simulink model "HumanDynamicsTest"  (R2021b)
settings: Solver=ode3  StartTime=0.0  StopTime=20  FixedStep=Ts  RelTol=1e-3
values from neighbouring files (symbols this model uses):
  B_m = diag(ones(1,dh.dof)) * 32    [setup_teleop.m]
  gravity = [0 0 9.81]'    [setup_robot.m]
  K_m = diag(ones(1,dh.dof)) * 22    [setup_teleop.m]
  KD_h = eye(dh.dof_task) * 2*z*wn    [setup_teleop.m]
  KP_h = eye(dh.dof_task) * wn^2    [setup_teleop.m]
  M_m = diag(ones(1,dh.dof)) * 22    [setup_teleop.m]
undefined symbols (not defined in the file or in its folder): conf, dh, Fm_A, Fm_B, x0
libraries: robotcorelib x1, simulink x1
settings Model: Creator=Sebastiano  LastModifiedBy=Sebastiano

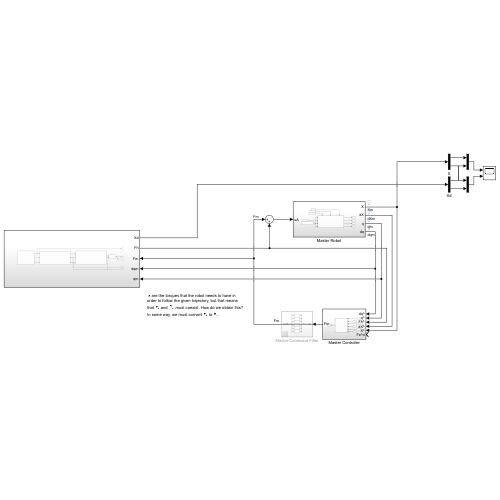
[thumbnail: Simulink's stored preview of the top-level diagram]
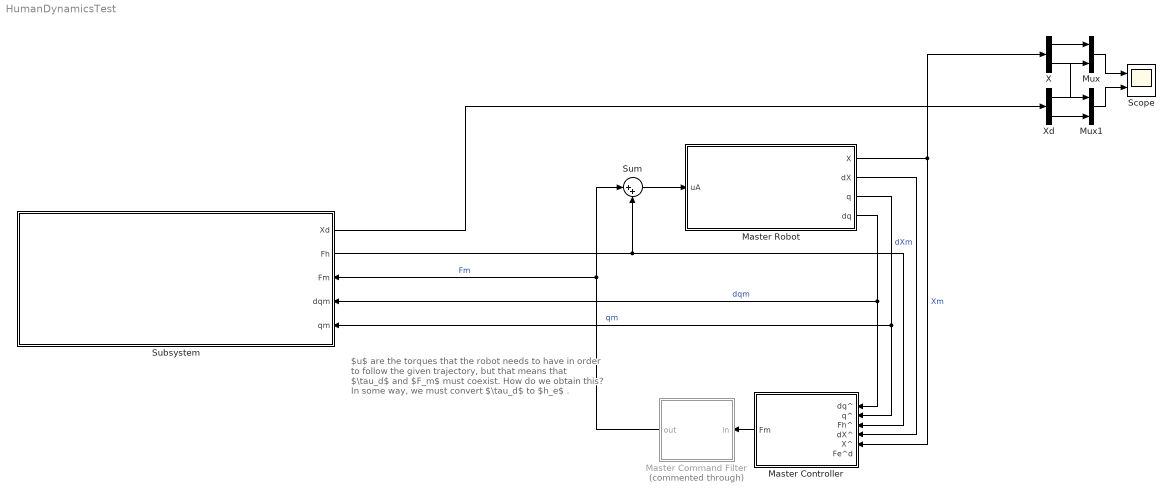
== system HumanDynamicsTest ==
  note: $u$ are the torques that the robot needs to have in order to follow the given trajectory, but that means that $\tau_d$ and $F_m$ must coexist. How do we obtain this? In some way, we must convert $\tau_d$ to $h_e$ .
  Master Command Filter : Subsystem  Commented=through
  Master Controller : Subsystem
  Master Robot : Subsystem
  Mux : Mux  Inputs=2
  Mux1 : Mux  Inputs=2
  Scope : Scope  NumInputPorts=2
  Subsystem : Subsystem
      settings: PortSchema="{\"entries\":[{\"content\":{\"sides\":[{\"content\":{\"connectorIds\":[]},\"type\":\"ConnectorPlacement.EquallySpacedRectSide\",\"uuid\":\"7778f5b7-85d4-4afc-857c-056ec77f7c35\"},{\"content\":{\"connectorIds\":[\"Out1\",\"Out2\",\"In1\",\"In2\",\"In3\"],\"side\":\"RIGHT\"},\"type\":\"ConnectorPlacement.EquallySpacedRectSide\",\"uuid\":\"4e6a4d83-f8e8-4554-84b1-926a6f2c9c17\"},{\"content\":{\"connectorIds\":[],\"side\":\"TOP\"},\"type\":\"ConnectorPlacement.EquallySpacedRectSide\",\"uuid\":\"7c53f63a-15b9-4620-895a-15c4690edfa5\"}]},\"type\":\"ConnectorPlacement.EquallySpacedConnector\",\"uuid\":\"f47fbd83-fa7b-4372-bf8b-e8c7b2e83c33\"}],\"packageUris\":[\"http://schema.mathworks.com/mf0/Connector/R2020b\"],\"version\":\"1.0\"}"
  Sum : Sum  Inputs=|++
  X : Demux  Outputs=2
  Xd : Demux  Outputs=2
  wires:
  Master Robot/3(q) -> Master Controller/2(q^), Subsystem/3(qm)  "qm"
  Master Robot/4(dq) -> Master Controller/1(dq^), Subsystem/2(dqm)  "dqm"
  Master Controller/1(Fm) -> Master Command Filter/1(in)
  Sum/1 -> Master Robot/1(uA)
  Master Robot/1(X) -> X/1, Master Controller/5(X^)  "Xm"
  Master Robot/2(dX) -> Master Controller/4(dX^)  "dXm"
  X/1 -> Mux/1
  Xd/1 -> Mux/2
  X/2 -> Mux1/1
  Xd/2 -> Mux1/2
  Mux/1 -> Scope/1
  Mux1/1 -> Scope/2
  Master Command Filter/1(out) -> Sum/1, Subsystem/1(Fm)  "Fm"
  Subsystem/2(Fh) -> Sum/2, Master Controller/3(Fh^)
  Subsystem/1(Xd) -> Xd/1

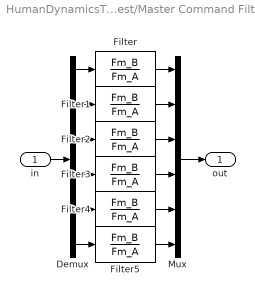
== system HumanDynamicsTest/Master Command Filter ==
  in : Inport
  Demux : Demux  Outputs=6
  Filter{,1..5} (6 alike) : TransferFcn  Numerator=Fm_B  Denominator=Fm_A
  Mux : Mux  Inputs=6
  out : Outport
  wires:
  Demux/4 -> Filter3/1
  Demux/6 -> Filter5/1
  Demux/2 -> Filter1/1
  Demux/5 -> Filter4/1
  Demux/1 -> Filter/1
  Demux/3 -> Filter2/1
  in/1 -> Demux/1
  Mux/1 -> out/1
  Filter/1 -> Mux/1
  Filter1/1 -> Mux/2
  Filter2/1 -> Mux/3
  Filter3/1 -> Mux/4
  Filter4/1 -> Mux/5
  Filter5/1 -> Mux/6

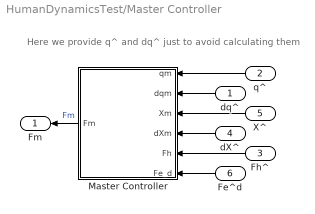
== system HumanDynamicsTest/Master Controller ==
  note: Here we provide q^ and dq^ just to avoid calculating them
  dq^ : Inport
  q^ : Inport  Port=2
  Fh^ : Inport  Port=3
  dX^ : Inport  Port=4
  X^ : Inport  Port=5
  Fe^d : Inport  Port=6
  Master Controller : MATLAB Function  TreatAsAtomicUnit=on
  Fm : Outport
  wires:
  Fh^/1 -> Master Controller/5(Fh)
  Fe^d/1 -> Master Controller/6(Fe_d)
  Master Controller/1(Fm) -> Fm/1  "Fm"
  X^/1 -> Master Controller/3(Xm)
  dX^/1 -> Master Controller/4(dXm)
  dq^/1 -> Master Controller/2(dqm)
  q^/1 -> Master Controller/1(qm)

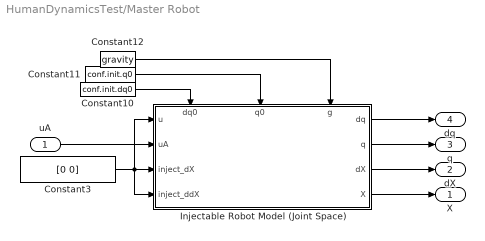
== system HumanDynamicsTest/Master Robot ==
  uA : Inport
  Constant10 : Constant  Value=conf.init.dq0
  Constant11 : Constant  Value=conf.init.q0
  Constant12 : Constant  Value=gravity
  Constant3 : Constant  Value=[0 0]
  Injectable Robot Model (Joint Space) : Subsystem
      settings: PortSchema="{\"entries\":[{\"content\":{\"sides\":[{\"content\":{\"connectorIds\":[\"In1\",\"In2\",\"In3\",\"In4\"]},\"type\":\"ConnectorPlacement.EquallySpacedRectSide\",\"uuid\":\"a8701c64-329e-4144-b882-ecf5d621aff2\"},{\"content\":{\"connectorIds\":[\"Out1\",\"Out2\",\"Out3\",\"Out4\"],\"side\":\"RIGHT\"},\"type\":\"ConnectorPlacement.EquallySpacedRectSide\",\"uuid\":\"4e168703-1cb9-438c-bc6b-9b2d7fbb809e\"},{\"content\":{\"connectorIds\":[\"In5\",\"In6\",\"In7\"],\"side\":\"TOP\"},\"type\":\"ConnectorPlacement.EquallySpacedRectSide\",\"uuid\":\"8fbcb29e-7fab-4224-b4ad-ee01c13d675a\"}]},\"type\":\"ConnectorPlacement.EquallySpacedConnector\",\"uuid\":\"fa721fab-1ce6-4fdf-95fa-8ada3ed2d65c\"}],\"packageUris\":[\"http://schema.mathworks.com/mf0/Connector/R2020b\"],\"version\":\"1.0\"}"
  X : Outport
  dX : Outport  Port=2
  q : Outport  Port=3
  dq : Outport  Port=4
  wires:
  Constant10/1 -> Injectable Robot Model (Joint Space)/5(dq0)
  Constant3/1 -> Injectable Robot Model (Joint Space)/1(u), Injectable Robot Model (Joint Space)/4(inject_ddX), Injectable Robot Model (Joint Space)/3(inject_dX)
  Constant11/1 -> Injectable Robot Model (Joint Space)/6(q0)
  Injectable Robot Model (Joint Space)/2(q) -> q/1
  Injectable Robot Model (Joint Space)/3(dX) -> dX/1
  Constant12/1 -> Injectable Robot Model (Joint Space)/7(g)
  Injectable Robot Model (Joint Space)/4(X) -> X/1
  Injectable Robot Model (Joint Space)/1(dq) -> dq/1
  uA/1 -> Injectable Robot Model (Joint Space)/2(uA)

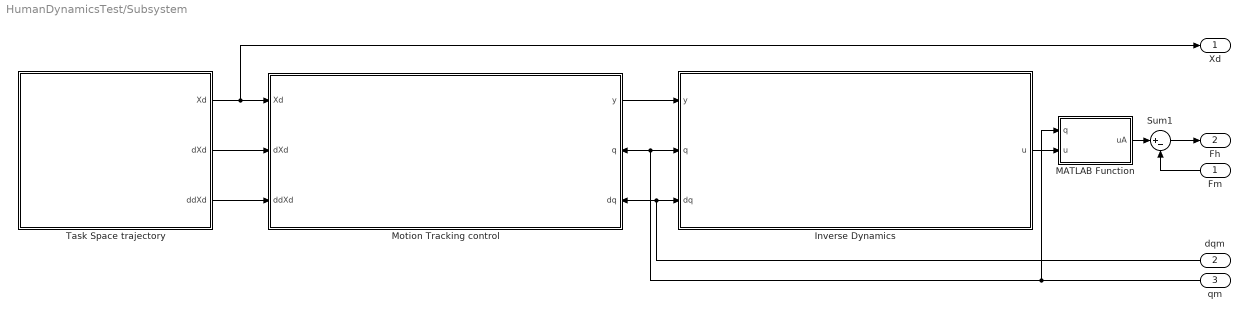
== system HumanDynamicsTest/Subsystem ==
  Fm : Inport
  dqm : Inport  Port=2
  qm : Inport  Port=3
  Inverse Dynamics : Subsystem
  MATLAB Function : MATLAB Function  TreatAsAtomicUnit=on
  Motion Tracking control : Subsystem
      settings: PortSchema="{\"entries\":[{\"content\":{\"sides\":[{\"content\":{\"connectorIds\":[\"In1\",\"In2\",\"In3\"]},\"type\":\"ConnectorPlacement.EquallySpacedRectSide\",\"uuid\":\"52575601-e286-4809-a30d-cedf982d9693\"},{\"content\":{\"connectorIds\":[\"Out1\",\"In4\",\"In5\"],\"side\":\"RIGHT\"},\"type\":\"ConnectorPlacement.EquallySpacedRectSide\",\"uuid\":\"ad2168cb-d0b7-4f4a-9914-0c84d01558f7\"},{\"content\":{\"connectorIds\":[],\"side\":\"TOP\"},\"type\":\"ConnectorPlacement.EquallySpacedRectSide\",\"uuid\":\"311024f8-e557-4a51-82a2-8dec63492c2b\"}]},\"type\":\"ConnectorPlacement.EquallySpacedConnector\",\"uuid\":\"f15c02cd-b134-4f17-b903-786a9234fd9d\"}],\"packageUris\":[\"http://schema.mathworks.com/mf0/Connector/R2020b\"],\"version\":\"1.0\"}"
  Sum1 : Sum  Inputs=|+-
  Task Space trajectory : Subsystem
  Xd : Outport
  Fh : Outport  Port=2
  wires:
  MATLAB Function/1(uA) -> Sum1/1
  Motion Tracking control/1(y) -> Inverse Dynamics/1(y)
  Task Space trajectory/2(dXd) -> Motion Tracking control/2(dXd)
  dqm/1 -> Motion Tracking control/5(dq), Inverse Dynamics/3(dq)
  Task Space trajectory/3(ddXd) -> Motion Tracking control/3(ddXd)
  Sum1/1 -> Fh/1
  qm/1 -> MATLAB Function/1(q), Inverse Dynamics/2(q), Motion Tracking control/4(q)
  Task Space trajectory/1(Xd) -> Xd/1, Motion Tracking control/1(Xd)
  Inverse Dynamics/1(u) -> MATLAB Function/2(u)
  Fm/1 -> Sum1/2

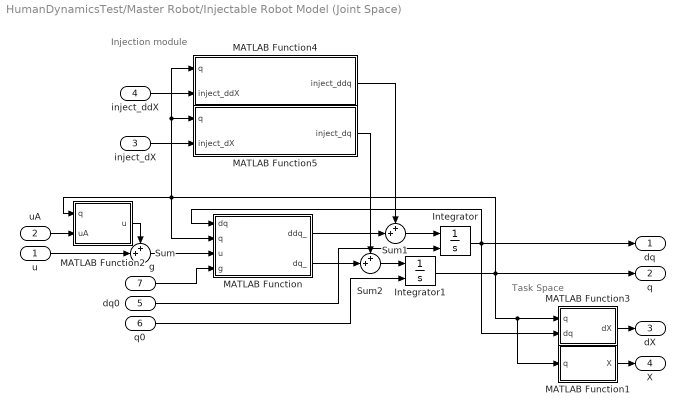
== system HumanDynamicsTest/Master Robot/Injectable Robot Model (Joint Space) ==
  note: Injection module
  note: Task Space
  u : Inport
  uA : Inport  Port=2
  inject_dX : Inport  Port=3
  inject_ddX : Inport  Port=4
  dq0 : Inport  Port=5
  q0 : Inport  Port=6
  g : Inport  Port=7
  Integrator : Integrator  InitialConditionSource=external  InitialCondition=x0
  Integrator1 : Integrator  InitialConditionSource=external  InitialCondition=x0
  MATLAB Function : MATLAB Function  TreatAsAtomicUnit=on
  MATLAB Function1 : MATLAB Function  TreatAsAtomicUnit=on
  MATLAB Function2 : MATLAB Function  TreatAsAtomicUnit=on
  MATLAB Function3 : MATLAB Function  TreatAsAtomicUnit=on
  MATLAB Function4 : MATLAB Function  TreatAsAtomicUnit=on
  MATLAB Function5 : MATLAB Function  TreatAsAtomicUnit=on
  Sum : Sum  Inputs=++|
  Sum1 : Sum  Inputs=++|
  Sum2 : Sum  Inputs=++|
  dq : Outport
  q : Outport  Port=2
  dX : Outport  Port=3
  X : Outport  Port=4
  wires:
  g/1 -> MATLAB Function/4(g)
  u/1 -> Sum/2
  dq0/1 -> Integrator/2
  Integrator1/1 -> q/1, MATLAB Function1/1(q), MATLAB Function3/1(q), MATLAB Function/2(q), MATLAB Function4/1(q), MATLAB Function5/1(q), MATLAB Function2/1(q)
  uA/1 -> MATLAB Function2/2(uA)
  MATLAB Function1/1(X) -> X/1
  Integrator/1 -> dq/1, MATLAB Function3/2(dq), MATLAB Function/1(dq)
  MATLAB Function3/1(dX) -> dX/1
  MATLAB Function2/1(u) -> Sum/1
  Sum/1 -> MATLAB Function/3(u)
  MATLAB Function/1(ddq_) -> Sum1/2
  q0/1 -> Integrator1/2
  Sum1/1 -> Integrator/1
  MATLAB Function/2(dq_) -> Sum2/2
  Sum2/1 -> Integrator1/1
  inject_ddX/1 -> MATLAB Function4/2(inject_ddX)
  inject_dX/1 -> MATLAB Function5/2(inject_dX)
  MATLAB Function4/1(inject_ddq) -> Sum1/1
  MATLAB Function5/1(inject_dq) -> Sum2/1

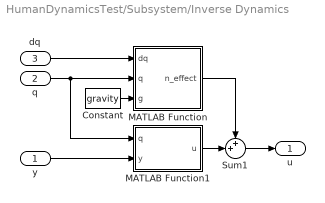
== system HumanDynamicsTest/Subsystem/Inverse Dynamics ==
  y : Inport
  q : Inport  Port=2
  dq : Inport  Port=3
  Constant : Constant  Value=gravity
  MATLAB Function : MATLAB Function  TreatAsAtomicUnit=on
  MATLAB Function1 : MATLAB Function  TreatAsAtomicUnit=on
  Sum1 : Sum  Inputs=++|
  u : Outport
  wires:
  dq/1 -> MATLAB Function/1(dq)
  MATLAB Function/1(n_effect) -> Sum1/1
  MATLAB Function1/1(u) -> Sum1/2
  q/1 -> MATLAB Function/2(q), MATLAB Function1/1(q)
  y/1 -> MATLAB Function1/2(y)
  Sum1/1 -> u/1
  Constant/1 -> MATLAB Function/3(g)

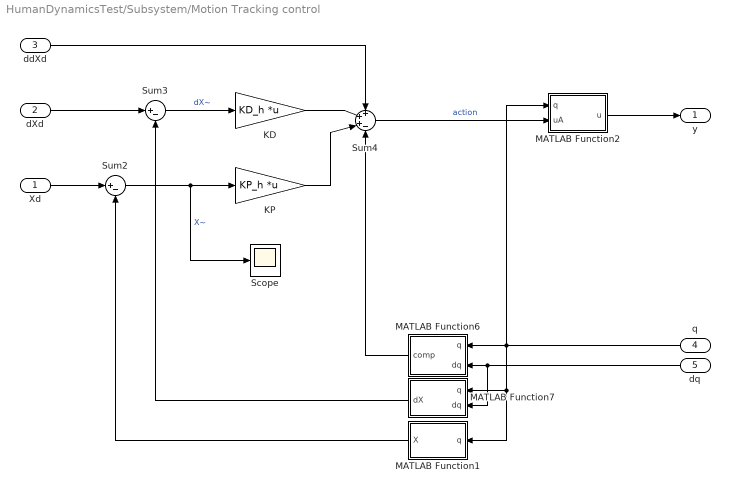
== system HumanDynamicsTest/Subsystem/Motion Tracking control ==
  Xd : Inport
  dXd : Inport  Port=2
  ddXd : Inport  Port=3
  q : Inport  Port=4
  dq : Inport  Port=5
  KD : Gain  Gain=KD_h  Multiplication=Matrix(K*u)
  KP : Gain  Gain=KP_h  Multiplication=Matrix(K*u)
  MATLAB Function1 : MATLAB Function  TreatAsAtomicUnit=on
  MATLAB Function2 : MATLAB Function  TreatAsAtomicUnit=on
  MATLAB Function6 : MATLAB Function  TreatAsAtomicUnit=on
  MATLAB Function7 : MATLAB Function  TreatAsAtomicUnit=on
  Scope : Scope
  Sum2 : Sum  Inputs=|+-
  Sum3 : Sum  Inputs=|+-
  Sum4 : Sum  Inputs=+++-
  y : Outport
  wires:
  MATLAB Function2/1(u) -> y/1
  dXd/1 -> Sum3/1
  ddXd/1 -> Sum4/1
  Xd/1 -> Sum2/1
  MATLAB Function7/1(dX) -> Sum3/2
  KP/1 -> Sum4/3
  Sum4/1 -> MATLAB Function2/2(uA)  "action"
  dq/1 -> MATLAB Function7/2(dq), MATLAB Function6/2(dq)
  q/1 -> MATLAB Function2/1(q), MATLAB Function6/1(q), MATLAB Function1/1(q), MATLAB Function7/1(q)
  Sum3/1 -> KD/1  "dX~"
  MATLAB Function1/1(X) -> Sum2/2
  MATLAB Function6/1(comp) -> Sum4/4
  Sum2/1 -> KP/1, Scope/1  "X~"
  KD/1 -> Sum4/2

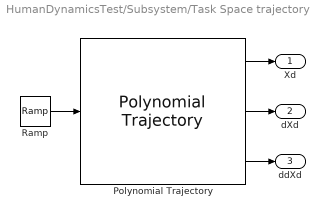
== system HumanDynamicsTest/Subsystem/Task Space trajectory ==
  Polynomial Trajectory : robotcorelib/Polynomial Trajectory  WaypointSource=Internal  Waypoints=[conf.init.x0 conf.init.x0+[0.1;0] conf.init.x0]  TimePoints=[ 0, 8, 16 ]  TimeInterval=[ 1, 4 ]  Method=Cubic Polynomial  ParameterSource=Internal  VelocityBoundaryCondition=zeros( 2, 3 )  AccelerationBoundaryCondition=zeros( 2, 5 )  SimulateUsing=Code generation
  Ramp : simulink/Sources/Ramp  slope=1  start=0  InitialOutput=0
  Xd : Outport
  dXd : Outport  Port=2
  ddXd : Outport  Port=3
  wires:
  Polynomial Trajectory/1 -> Xd/1
  Polynomial Trajectory/2 -> dXd/1
  Ramp/1 -> Polynomial Trajectory/1
  Polynomial Trajectory/3 -> ddXd/1

== matlab function HumanDynamicsTest/Master Robot/Injectable Robot Model (Joint Space)/MATLAB Function4 ==
  data: q input size=dh.dof; inject_ddq output size=dh.dof; inject_ddX input size=2; dh parameter
function inject_ddq = get_inject_ddq(q, inject_ddX, dh)
    JA = JA_rne(dh, q);
    inject_ddq = pinv(JA) * inject_ddX;
end

== matlab function HumanDynamicsTest/Master Robot/Injectable Robot Model (Joint Space)/MATLAB Function5 ==
  data: q input size=dh.dof; inject_dq output size=dh.dof; inject_dX input size=2; dh parameter
function inject_dq = get_inject_dq(q, inject_dX, dh)
    JA = JA_rne(dh, q);
    inject_dq = pinv(JA) * inject_dX;
end

== matlab function HumanDynamicsTest/Subsystem/Motion Tracking control/MATLAB Function2 ==
  data: dh parameter; u output; q input; uA input
function u = JAinv(dh, q, uA)
    JA = JA_rne(dh, q);
    u = pinv(JA)*uA;
end

== matlab function HumanDynamicsTest/Subsystem/Motion Tracking control/MATLAB Function1 ==
  data: X output; q input; dh parameter
function X = K(q, dh)
    X = K_rne(dh, q);
end

== matlab function HumanDynamicsTest/Subsystem/Motion Tracking control/MATLAB Function6 ==
  data: q input size=dh.dof; dq input size=dh.dof; comp output size=dh.dof_task; dh parameter
function comp = JAD(q,dq, dh)
    % little theoretic insert:
    % since  TA*JA = J  we have
    %   (TA*JA)' = (J)'
    %   TAD*JA +  TA*JAD = JD
    %   JAD = TA \ (JD - TAD*JA)
    % but we have JDdq! fortunally, since we actually want JAD*dq we have
    %   JAD*dq = TA \ (JD - TAD*JA)*dq
    %          = TA \ (JD*dq - TAD*JA*dq)
    %          = TA \ (JDdq - TAD*dX)

    JA = JA_rne(dh,q);
    TA = TA_rne(dh,q);
    TAD = TAD_rne(dh,q,dq);
    JDdq = JDdq_rne(dh,q,dq);

    comp = pinv(TA) * (JDdq - TAD*JA*dq);
end

== matlab function HumanDynamicsTest/Subsystem/Motion Tracking control/MATLAB Function7 ==
  data: dh parameter; dX output; q input; dq input
function dX = JA(dh, q, dq)
    dX = JA_rne(dh, q)*dq;
end

== matlab function HumanDynamicsTest/Subsystem/Inverse Dynamics/MATLAB Function ==
  data: dq input size=dh.dof; q input size=dh.dof; n_effect output size=dh.dof; g input size=3; dh parameter
function n_effect = n(dq,q, g, dh)
    n_effect = C_rne(dh,q,dq)*dq + G_rne(dh,q,g);
end

== matlab function HumanDynamicsTest/Subsystem/MATLAB Function ==
  data: q input size=dh.dof; u input; uA output; dh parameter
function uA = JAinvT(q,u, dh)
    uA = pinv(JA_rne(dh, q))' * u;
end

== matlab function HumanDynamicsTest/Master Robot/Injectable Robot Model (Joint Space)/MATLAB Function ==
  data ddq_ settings: updateMethod=SF_CONTINUOUS_TIME_DATA
  data dq_ settings: updateMethod=SF_CONTINUOUS_TIME_DATA
  data dq settings: updateMethod=SF_CONTINUOUS_TIME_DATA
  data q settings: updateMethod=SF_CONTINUOUS_TIME_DATA
  data u settings: updateMethod=SF_CONTINUOUS_TIME_DATA
  data: ddq_ output size=dh.dof; dq_ output size=dh.dof; dq input size=dh.dof; q input size=dh.dof; u input size=dh.dof; g input size=3; dh parameter
function [ddq_, dq_]  = RobotSystem(dq, q, u, g, dh)
    
    % compute dynamics
    B = B_rne(dh, q);
    C = C_rne(dh, q, dq);
    G = G_rne(dh, q, g);

    dq_ = dq(1:dh.dof);

    ddq = B \ (u - C*dq - G);
    ddq_ = ddq(1:dh.dof);
end

== matlab function HumanDynamicsTest/Master Robot/Injectable Robot Model (Joint Space)/MATLAB Function1 ==
  data: X output; q input; dh parameter
function X = K(q, dh)
    X = K_rne(dh, q);
end

== matlab function HumanDynamicsTest/Subsystem/Inverse Dynamics/MATLAB Function1 ==
  data: q input size=dh.dof; u output size=dh.dof; y input size=dh.dof; dh parameter
function u = B(q,y, dh)
    u = B_rne(dh,q)*y;
end

== matlab function HumanDynamicsTest/Master Robot/Injectable Robot Model (Joint Space)/MATLAB Function2 ==
  data: q input; uA input; u output; dh parameter
function u = JAT(q,uA, dh)
    u = JA_rne(dh,q)' * uA;
end

== matlab function HumanDynamicsTest/Master Robot/Injectable Robot Model (Joint Space)/MATLAB Function3 ==
  data: dh parameter; dX output; q input; dq input
function dX = JA(dh, q, dq)
    dX = JA_rne(dh, q)*dq;
end

== matlab function HumanDynamicsTest/Master Controller/Master Controller ==
  data: dh parameter; qm input size=dh.dof; dqm input size=dh.dof; Xm input size=2; Fm output size=2; dXm input size=2; Fh input size=2; Fe_d input size=2; gravity parameter size=3; M_m parameter size=[2,2]; B_m parameter size=[2,2]; K_m parameter size=[2,2]
function Fm = Cm(dh,qm,dqm, Xm,dXm, Fh,Fe_d,gravity, M_m,B_m,K_m)
    
    BA = BA_rne(dh, qm);
    CAdX = CAdX_rne(dh, qm, dqm);  % we can use CAdX instead of CA*dX since here dq and dX have the same meaning
    GA = GA_rne(dh, qm, gravity);

    % inner impedance controller
    vm = M_m \ (-B_m*dXm - K_m*Xm + Fh - Fe_d);
    % outer decoupling/linearization controller
    Fm = BA*vm + CAdX + GA - Fh;
end
